simulink model "linear_flight_controller_payload"  (R2020a)
settings: Solver=FixedStepAuto  StartTime=0.0  StopTime=50  FixedStep=0.005  RelTol=1e-3
InitFcn:
  | flight_controller_payload_setup % Script to setup workspace
values from neighbouring files (symbols this model uses):
  C_Dx = 0.2    [PID_design_setup.m]    (also in flight_controller_payload_setup.m)
  C_Dz = 0.2    [PID_design_setup.m]    (also in flight_controller_payload_setup.m)
  C_px = 0.05    [flight_controller_payload_setup.m]
  C_pz = 0.05    [flight_controller_payload_setup.m]
  cbeta = 0.05    [flight_controller_payload_setup.m]
  dtheta_sp_max = 120*pi/180    (= 2.09439510239)    [flight_controller_payload_setup.m]
  dtheta_sp_min = -120*pi/180    (= -2.09439510239)    [flight_controller_payload_setup.m]
  dx_sp_max = 12    [flight_controller_payload_setup.m]
  dx_sp_min = -12    [flight_controller_payload_setup.m]
  dz_sp_max = 12    [flight_controller_payload_setup.m]
  dz_sp_min = -12    [flight_controller_payload_setup.m]
  g = -9.81    [PID_design_setup.m]    (also in flight_controller_payload_setup.m)
  I_yy = 0.235    [PID_design_setup.m]    (also in flight_controller_payload_setup.m)
  ki_dtheta = kp_dtheta*z_c    (= 0.1)    [PID_design_setup.m]
  kp_dtheta = 10^(K_dB/20)    [PID_design_setup.m]
  l = 1    [flight_controller_payload_setup.m]
  M = 4.5    [PID_design_setup.m]    (also in flight_controller_payload_setup.m)
  m = 2    [flight_controller_payload_setup.m]
  MM = [-1, 1 ... (first row only)    [flight_controller_payload_setup.m]    (also in flight_controller_setup.m = [-1/sqrt(2), -1)
  N_dtheta = Inf    (= inf)    [flight_controller_payload_setup.m]
  N_dx = 5*2*pi    (= 31.4159265359)    [flight_controller_payload_setup.m]
  N_dz = 5*2*pi    (= 31.4159265359)    [flight_controller_payload_setup.m]
  r = 0.49*1/sqrt(2)    [PID_design_setup.m]    (also in flight_controller_payload_setup.m)
  rho = 1.225    [PID_design_setup.m]    (also in flight_controller_payload_setup.m)
  sigma = 0    [flight_controller_payload_setup.m]
  tau = 0.07    [PID_design_setup.m]    (also in flight_controller_payload_setup.m)
  theta_sp_max = 30*pi/180    (= 0.523598775598)    [flight_controller_payload_setup.m]
  theta_sp_min = -30*pi/180    (= -0.523598775598)    [flight_controller_payload_setup.m]
  Ts_excite = 0    [flight_controller_payload_setup.m]
  Ts_mpc = 0.03    [flight_controller_payload_setup.m]
  u0 = -0.5*M*g*[1; 1]    [flight_controller_payload_setup.m]
  var_excite = 0    [flight_controller_payload_setup.m]
  x0 = zeros(nx,1)    [flight_controller_payload_setup.m]    (also in flight_controller_setup.m = zeros(6,1))
  x0_no_load = zeros(6,1)    [flight_controller_payload_setup.m]
undefined symbols (not defined in the file or in its folder): A_lin, B_lin, kd_dtheta, kd_dx, kd_dz, ki_dx, ki_dz, kp_dx, kp_dz, kp_theta, kp_x, kp_z
libraries: simulink x26, dspstat3 x8, mpclib x2
(part 3 of 3)

== system linear_flight_controller_payload/state space WITHOUT payload1/Angular rate controller1 ==
  note: PID to use auto tuning from simulink
  dtheta_sp : Inport
  X : Inport  Port=2
  Demux1 : Demux  Outputs=6
  Derivative : Derivative
  Gain : Gain  Gain=kd_dtheta
  I : Gain  Gain=ki_dtheta
  Integrator Limited : Integrator  LimitOutput=on  UpperSaturationLimit=10  LowerSaturationLimit=-10
  Low Pass Filter : TransferFcn  Denominator=[1/N_dtheta, 1]
  P : Gain  Gain=kp_dtheta
  PID Omega Controller : simulink/Continuous/PID Controller  Commented=on  Controller=PID  Form=Parallel  TimeDomain=Continuous-time  UseExternalTs=off  SampleTime=-1  IntegratorMethod=Forward Euler  FilterMethod=Forward Euler  ControllerParametersSource=internal  P=kp_dtheta  I=ki_dtheta  D=kd_dtheta  UseFilter=on  N=N_dtheta  TunerSelectOption=Transfer Function Based (PID Tuner App)  InitialConditionSource=internal  InitialConditionForIntegrator=0  InitialConditionForFilter=0  DifferentiatorICPrevScaledInput=0  ExternalReset=none  TrackingMode=off  Kt=1  LimitOutput=off  UpperSaturationLimit=inf  LowerSaturationLimit=-inf  LinearizeAsGain=on  AntiWindupMode=none  Kb=1  POutMin=[]  POutMax=[]  IOutMin=[]  IOutMax=[]  DOutMin=[]  DOutMax=[]  NOutMin=[]  NOutMax=[]  SumOutMin=[]  SumOutMax=[]  SaturationOutMin=[]  SaturationOutMax=[]  PParamMin=[]  PParamMax=[]  IParamMin=[]  IParamMax=[]  DParamMin=[]  DParamMax=[]  NParamMin=[]  NParamMax=[]  KbParamMin=[]  KbParamMax=[]  KtParamMin=[]  KtParamMax=[]  KbOutMin=[]  KbOutMax=[]  KtOutMin=[]  KtOutMax=[]  IntegratorOutMin=[]  IntegratorOutMax=[]  FilterOutMin=[]  FilterOutMax=[]  SumI1OutMin=[]  SumI1OutMax=[]  SumI2OutMin=[]  SumI2OutMax=[]  SumI3OutMin=[]  SumI3OutMax=[]  SumI4OutMin=[]  SumI4OutMax=[]  SumDOutMin=[]  SumDOutMax=[]  DifferentiatorOutMin=[]  DifferentiatorOutMax=[]  FilterDiffOutCoefMin=[]  FilterDiffOutCoefMax=[]  ReciprocalOutMin=[]  ReciprocalOutMax=[]  SumDenOutMin=[]  SumDenOutMax=[]  SumNumOutMin=[]  SumNumOutMax=[]  DivideOutMin=[]  DivideOutMax=[]  UdiffTsProdOutMin=[]  UdiffTsProdOutMax=[]  NTsProdOutMin=[]  NTsProdOutMax=[]  UintegralTsProdOutMin=[]  UintegralTsProdOutMax=[]  UngainTsProdOutMin=[]  UngainTsProdOutMax=[]  IntegratorContinuousStateAttributes=''  IntegratorStateMustResolveToSignalObject=off  IntegratorRTWStateStorageClass=Auto  FilterContinuousStateAttributes=''  FilterStateMustResolveToSignalObject=off  FilterRTWStateStorageClass=Auto  ParallelPVariant=InternalParameters  IdealPVariant=Disabled  IVariant=InternalParameters  DVariant=InternalParameters  IntegratorVariant=Continuous  SatVariant=Disabled  AWVariant=Passthrough  PCopyVariant=Disabled  TRVariant=Disabled  FdbkBlocksVariant=Forward  IdealPFdbkVariant=Disabled  SatFdbkVariant=Disabled  DerivativeFilterVariant=ContFilter  NVariant=InternalParameters  NCopyVariant=Disabled  FilterICVariant=InternalICsFilter  IntegratorICVariant=InternalICs  ExternalResetVariant=Disabled  TRSumVariant=Passthrough  SumFdbkVariant=Disabled  SumVariant=Sum_PID  TsampFilterVariant=InternalTs  TsampNgainVariant=Passthrough  TsampIntegralVariant=Passthrough
  Sum : Sum  Inputs=|+-
  Sum1 : Sum  Inputs=++-
  Sum2 : Sum  Inputs=++|
  delta_E : Outport
  wires:
  dtheta_sp/1 -> Sum/1
  Sum/1 -> P/1, Integrator Limited/1, PID Omega Controller/1
  Integrator Limited/1 -> I/1
  Derivative/1 -> Gain/1
  I/1 -> Sum1/2
  P/1 -> Sum1/1
  Gain/1 -> Sum1/3
  Sum1/1 -> Sum2/2
  Sum2/1 -> delta_E/1
  PID Omega Controller/1 -> Sum2/1
  Low Pass Filter/1 -> Derivative/1
  X/1 -> Demux1/1
  Demux1/6 -> Low Pass Filter/1, Sum/2  "dtheta"

== system linear_flight_controller_payload/state space WITHOUT payload1/Motor Mixing Algorithm1 ==
  delta_E : Inport
  delta_T : Inport  Port=2
  Mixing Matrix : Gain  Gain=MM  Multiplication=Matrix(K*u)
  Mux : Mux  Inputs=2
  Signal Specification : SignalSpecification  Dimensions=[2, 1]
  u : Outport  LockScale=on
  wires:
  delta_T/1 -> Mux/2
  delta_E/1 -> Mux/1
  Mixing Matrix/1 -> u/1
  Mux/1 -> Signal Specification/1
  Signal Specification/1 -> Mixing Matrix/1

== system linear_flight_controller_payload/state space WITHOUT payload1/Plant WITHOUT payload ==
  u : Inport  PortDimensions=[2, 1]
  Integrator : Integrator  Commented=on  InitialCondition=x0_no_load
  MATLAB Function1 : MATLAB Function  Commented=on  TreatAsAtomicUnit=on
  Motors : Subsystem
  Signal Specification : SignalSpecification  Dimensions=2
  State-Space : StateSpace  A=A_lin  B=B_lin  C=eye(6)  D=zeros(size(B_lin))  InitialCondition=zeros(6,1)
  parameters : Subsystem  Commented=on
  x : Outport
  wires:
  Motors/1(T) -> Signal Specification/1
  u/1 -> Motors/1(T_r)
  ? -> MATLAB Function1/2(u)
  Integrator/1 -> MATLAB Function1/1(x)
  parameters/1(parameters) -> MATLAB Function1/3(params)
  MATLAB Function1/1(dx) -> Integrator/1
  Signal Specification/1 -> State-Space/1
  State-Space/1 -> x/1

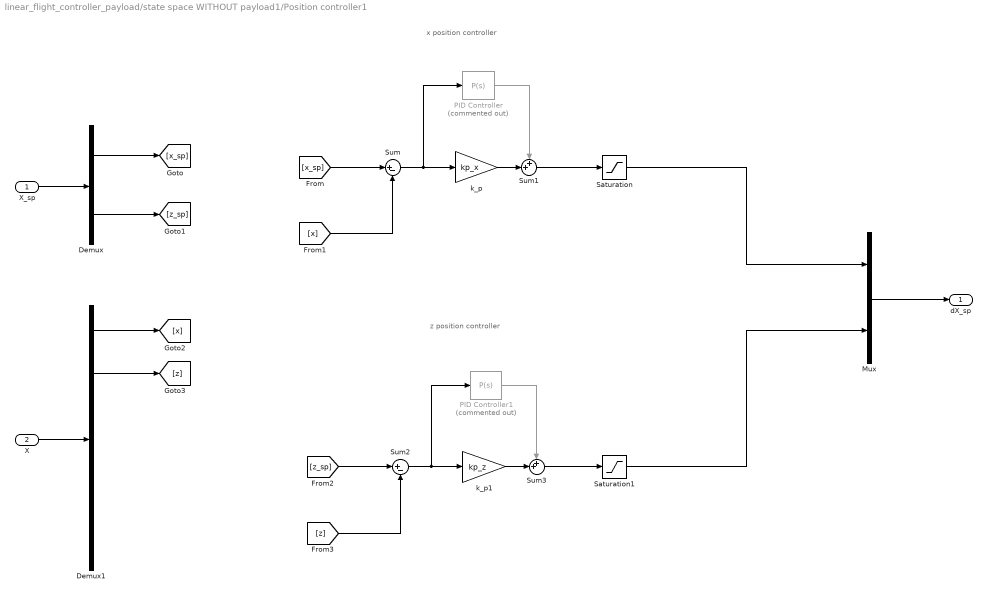
== system linear_flight_controller_payload/state space WITHOUT payload1/Position controller1 ==
  note: x position controller
  note: z position controller
  X_sp : Inport
  X : Inport  Port=2
  Demux : Demux  Outputs=2
  Demux1 : Demux  Outputs=6
  Mux : Mux  Inputs=2
  PID Controller : simulink/Continuous/PID Controller  Commented=on  Controller=P  Form=Parallel  TimeDomain=Continuous-time  UseExternalTs=off  SampleTime=-1  IntegratorMethod=Forward Euler  FilterMethod=Forward Euler  ControllerParametersSource=internal  P=20  I=1  D=0  UseFilter=on  N=100  TunerSelectOption=Transfer Function Based (PID Tuner App)  InitialConditionSource=internal  InitialConditionForIntegrator=0  InitialConditionForFilter=0  DifferentiatorICPrevScaledInput=0  ExternalReset=none  TrackingMode=off  Kt=1  LimitOutput=off  UpperSaturationLimit=inf  LowerSaturationLimit=-inf  LinearizeAsGain=on  AntiWindupMode=none  Kb=1  POutMin=[]  POutMax=[]  IOutMin=[]  IOutMax=[]  DOutMin=[]  DOutMax=[]  NOutMin=[]  NOutMax=[]  SumOutMin=[]  SumOutMax=[]  SaturationOutMin=[]  SaturationOutMax=[]  PParamMin=[]  PParamMax=[]  IParamMin=[]  IParamMax=[]  DParamMin=[]  DParamMax=[]  NParamMin=[]  NParamMax=[]  KbParamMin=[]  KbParamMax=[]  KtParamMin=[]  KtParamMax=[]  KbOutMin=[]  KbOutMax=[]  KtOutMin=[]  KtOutMax=[]  IntegratorOutMin=[]  IntegratorOutMax=[]  FilterOutMin=[]  FilterOutMax=[]  SumI1OutMin=[]  SumI1OutMax=[]  SumI2OutMin=[]  SumI2OutMax=[]  SumI3OutMin=[]  SumI3OutMax=[]  SumI4OutMin=[]  SumI4OutMax=[]  SumDOutMin=[]  SumDOutMax=[]  DifferentiatorOutMin=[]  DifferentiatorOutMax=[]  FilterDiffOutCoefMin=[]  FilterDiffOutCoefMax=[]  ReciprocalOutMin=[]  ReciprocalOutMax=[]  SumDenOutMin=[]  SumDenOutMax=[]  SumNumOutMin=[]  SumNumOutMax=[]  DivideOutMin=[]  DivideOutMax=[]  UdiffTsProdOutMin=[]  UdiffTsProdOutMax=[]  NTsProdOutMin=[]  NTsProdOutMax=[]  UintegralTsProdOutMin=[]  UintegralTsProdOutMax=[]  UngainTsProdOutMin=[]  UngainTsProdOutMax=[]  IntegratorContinuousStateAttributes=''  IntegratorStateMustResolveToSignalObject=off  IntegratorRTWStateStorageClass=Auto  FilterContinuousStateAttributes=''  FilterStateMustResolveToSignalObject=off  FilterRTWStateStorageClass=Auto  ParallelPVariant=InternalParameters  IdealPVariant=Disabled  IVariant=Disabled  DVariant=Disabled  IntegratorVariant=Disabled  SatVariant=Disabled  AWVariant=Disabled  PCopyVariant=Disabled  TRVariant=Disabled  FdbkBlocksVariant=Forward  IdealPFdbkVariant=Disabled  SatFdbkVariant=Disabled  DerivativeFilterVariant=Disabled  NVariant=Disabled  NCopyVariant=Disabled_SignalSpec  FilterICVariant=Disabled  IntegratorICVariant=Disabled  ExternalResetVariant=Disabled  TRSumVariant=Passthrough  SumFdbkVariant=Disabled  SumVariant=Passthrough_P  TsampFilterVariant=InternalTs  TsampNgainVariant=Passthrough  TsampIntegralVariant=Disabled_SignalSpec
  PID Controller1 : simulink/Continuous/PID Controller  Commented=on  Controller=P  Form=Parallel  TimeDomain=Continuous-time  UseExternalTs=off  SampleTime=-1  IntegratorMethod=Forward Euler  FilterMethod=Forward Euler  ControllerParametersSource=internal  P=1  I=1  D=0  UseFilter=on  N=100  TunerSelectOption=Transfer Function Based (PID Tuner App)  InitialConditionSource=internal  InitialConditionForIntegrator=0  InitialConditionForFilter=0  DifferentiatorICPrevScaledInput=0  ExternalReset=none  TrackingMode=off  Kt=1  LimitOutput=off  UpperSaturationLimit=inf  LowerSaturationLimit=-inf  LinearizeAsGain=on  AntiWindupMode=none  Kb=1  POutMin=[]  POutMax=[]  IOutMin=[]  IOutMax=[]  DOutMin=[]  DOutMax=[]  NOutMin=[]  NOutMax=[]  SumOutMin=[]  SumOutMax=[]  SaturationOutMin=[]  SaturationOutMax=[]  PParamMin=[]  PParamMax=[]  IParamMin=[]  IParamMax=[]  DParamMin=[]  DParamMax=[]  NParamMin=[]  NParamMax=[]  KbParamMin=[]  KbParamMax=[]  KtParamMin=[]  KtParamMax=[]  KbOutMin=[]  KbOutMax=[]  KtOutMin=[]  KtOutMax=[]  IntegratorOutMin=[]  IntegratorOutMax=[]  FilterOutMin=[]  FilterOutMax=[]  SumI1OutMin=[]  SumI1OutMax=[]  SumI2OutMin=[]  SumI2OutMax=[]  SumI3OutMin=[]  SumI3OutMax=[]  SumI4OutMin=[]  SumI4OutMax=[]  SumDOutMin=[]  SumDOutMax=[]  DifferentiatorOutMin=[]  DifferentiatorOutMax=[]  FilterDiffOutCoefMin=[]  FilterDiffOutCoefMax=[]  ReciprocalOutMin=[]  ReciprocalOutMax=[]  SumDenOutMin=[]  SumDenOutMax=[]  SumNumOutMin=[]  SumNumOutMax=[]  DivideOutMin=[]  DivideOutMax=[]  UdiffTsProdOutMin=[]  UdiffTsProdOutMax=[]  NTsProdOutMin=[]  NTsProdOutMax=[]  UintegralTsProdOutMin=[]  UintegralTsProdOutMax=[]  UngainTsProdOutMin=[]  UngainTsProdOutMax=[]  IntegratorContinuousStateAttributes=''  IntegratorStateMustResolveToSignalObject=off  IntegratorRTWStateStorageClass=Auto  FilterContinuousStateAttributes=''  FilterStateMustResolveToSignalObject=off  FilterRTWStateStorageClass=Auto  ParallelPVariant=InternalParameters  IdealPVariant=Disabled  IVariant=Disabled  DVariant=Disabled  IntegratorVariant=Disabled  SatVariant=Disabled  AWVariant=Disabled  PCopyVariant=Disabled  TRVariant=Disabled  FdbkBlocksVariant=Forward  IdealPFdbkVariant=Disabled  SatFdbkVariant=Disabled  DerivativeFilterVariant=Disabled  NVariant=Disabled  NCopyVariant=Disabled_SignalSpec  FilterICVariant=Disabled  IntegratorICVariant=Disabled  ExternalResetVariant=Disabled  TRSumVariant=Passthrough  SumFdbkVariant=Disabled  SumVariant=Passthrough_P  TsampFilterVariant=InternalTs  TsampNgainVariant=Passthrough  TsampIntegralVariant=Disabled_SignalSpec
  Saturation : Saturate  UpperLimit=dx_sp_max  LowerLimit=dx_sp_min
  Saturation1 : Saturate  UpperLimit=dz_sp_max  LowerLimit=dz_sp_min
  Sum : Sum  Inputs=|+-
  Sum1 : Sum  Inputs=++|
  Sum2 : Sum  Inputs=|+-
  Sum3 : Sum  Inputs=++|
  k_p : Gain  Gain=kp_x
  k_p1 : Gain  Gain=kp_z
  dX_sp : Outport
  wires:
  Sum/1 -> PID Controller/1, k_p/1
  k_p/1 -> Sum1/2
  PID Controller/1 -> Sum1/1
  X_sp/1 -> Demux/1
  Demux/2 -> [z_sp]
  Demux/1 -> [x_sp]
  X/1 -> Demux1/1
  Demux1/1 -> [x]
  Demux1/2 -> [z]
  [x_sp] -> Sum/1
  [x] -> Sum/2
  Sum2/1 -> PID Controller1/1, k_p1/1
  [z] -> Sum2/2
  [z_sp] -> Sum2/1
  PID Controller1/1 -> Sum3/1
  k_p1/1 -> Sum3/2
  Mux/1 -> dX_sp/1
  Sum1/1 -> Saturation/1
  Sum3/1 -> Saturation1/1
  Saturation1/1 -> Mux/2
  Saturation/1 -> Mux/1

== system linear_flight_controller_payload/state space WITHOUT payload1/Subsystem1 ==
  X : Inport
  Demux : Demux  Outputs=6
  theta : Outport
  wires:
  X/1 -> Demux/1
  Demux/3 -> theta/1

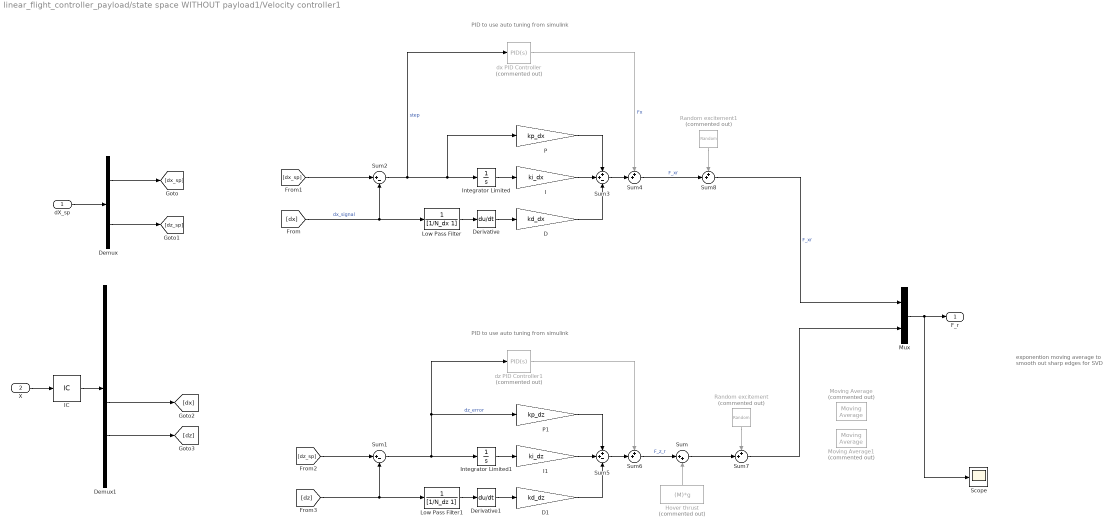
== system linear_flight_controller_payload/state space WITHOUT payload1/Velocity controller1 ==
  note: exponention moving average
      | to smooth out sharp edges for SVD
  note: PID to use auto tuning from simulink
  note: PID to use auto tuning from simulink
  dX_sp : Inport
  X : Inport  Port=2
  D : Gain  Gain=kd_dx
  D1 : Gain  Gain=kd_dz
  Demux : Demux  Outputs=2
  Demux1 : Demux  Outputs=6
  Derivative : Derivative
  Derivative1 : Derivative
  Hover thrust : Constant  Commented=on  Value=(M)*g
  I : Gain  Gain=ki_dx
  I1 : Gain  Gain=ki_dz
  IC : InitialCondition  Value=x0_no_load
  Integrator Limited : Integrator  LimitOutput=on  UpperSaturationLimit=10  LowerSaturationLimit=-10
  Integrator Limited1 : Integrator  LimitOutput=on  UpperSaturationLimit=10  LowerSaturationLimit=-10
  Low Pass Filter : TransferFcn  Denominator=[1/N_dx 1]
  Low Pass Filter1 : TransferFcn  Denominator=[1/N_dz 1]
  Moving Average : dspstat3/Moving Average  Commented=on  Method=Exponential weighting  ForgettingFactorPort=off  SpecifyWindowLength=on  WindowLength=4  ForgettingFactor=lambda  SimulateUsing=Code generation
  Moving Average1 : dspstat3/Moving Average  Commented=on  Method=Exponential weighting  ForgettingFactorPort=off  SpecifyWindowLength=on  WindowLength=4  ForgettingFactor=lambda  SimulateUsing=Code generation
  Mux : Mux  Inputs=2
  P : Gain  Gain=kp_dx
  P1 : Gain  Gain=kp_dz
  Random excitement : RandomNumber  Commented=on  Variance=var_excite  SampleTime=Ts_excite
  Random excitement1 : RandomNumber  Commented=on  Variance=var_excite  Seed=1  SampleTime=Ts_excite
  Scope : Scope
  Sum : Sum  Inputs=|++
  Sum1 : Sum  Inputs=|+-
  Sum2 : Sum  Inputs=|+-
  Sum3 : Sum  Inputs=++-
  Sum{4,6..8} (4 alike) : Sum  Inputs=++|
  Sum5 : Sum  Inputs=++-
  dx PID Controller : simulink/Continuous/PID Controller  Commented=on  Controller=PID  Form=Parallel  TimeDomain=Continuous-time  UseExternalTs=off  SampleTime=-1  IntegratorMethod=Forward Euler  FilterMethod=Forward Euler  ControllerParametersSource=internal  P=kp_dx  I=ki_dx  D=kd_dx  UseFilter=on  N=N_dx  TunerSelectOption=Transfer Function Based (PID Tuner App)  InitialConditionSource=internal  InitialConditionForIntegrator=0  InitialConditionForFilter=0  DifferentiatorICPrevScaledInput=0  ExternalReset=none  TrackingMode=off  Kt=1  LimitOutput=off  UpperSaturationLimit=inf  LowerSaturationLimit=-inf  LinearizeAsGain=on  AntiWindupMode=none  Kb=1  POutMin=[]  POutMax=[]  IOutMin=[]  IOutMax=[]  DOutMin=[]  DOutMax=[]  NOutMin=[]  NOutMax=[]  SumOutMin=[]  SumOutMax=[]  SaturationOutMin=[]  SaturationOutMax=[]  PParamMin=[]  PParamMax=[]  IParamMin=[]  IParamMax=[]  DParamMin=[]  DParamMax=[]  NParamMin=[]  NParamMax=[]  KbParamMin=[]  KbParamMax=[]  KtParamMin=[]  KtParamMax=[]  KbOutMin=[]  KbOutMax=[]  KtOutMin=[]  KtOutMax=[]  IntegratorOutMin=[]  IntegratorOutMax=[]  FilterOutMin=[]  FilterOutMax=[]  SumI1OutMin=[]  SumI1OutMax=[]  SumI2OutMin=[]  SumI2OutMax=[]  SumI3OutMin=[]  SumI3OutMax=[]  SumI4OutMin=[]  SumI4OutMax=[]  SumDOutMin=[]  SumDOutMax=[]  DifferentiatorOutMin=[]  DifferentiatorOutMax=[]  FilterDiffOutCoefMin=[]  FilterDiffOutCoefMax=[]  ReciprocalOutMin=[]  ReciprocalOutMax=[]  SumDenOutMin=[]  SumDenOutMax=[]  SumNumOutMin=[]  SumNumOutMax=[]  DivideOutMin=[]  DivideOutMax=[]  UdiffTsProdOutMin=[]  UdiffTsProdOutMax=[]  NTsProdOutMin=[]  NTsProdOutMax=[]  UintegralTsProdOutMin=[]  UintegralTsProdOutMax=[]  UngainTsProdOutMin=[]  UngainTsProdOutMax=[]  IntegratorContinuousStateAttributes=''  IntegratorStateMustResolveToSignalObject=off  IntegratorRTWStateStorageClass=Auto  FilterContinuousStateAttributes=''  FilterStateMustResolveToSignalObject=off  FilterRTWStateStorageClass=Auto  ParallelPVariant=InternalParameters  IdealPVariant=Disabled  IVariant=InternalParameters  DVariant=InternalParameters  IntegratorVariant=Continuous  SatVariant=Disabled  AWVariant=Passthrough  PCopyVariant=Disabled  TRVariant=Disabled  FdbkBlocksVariant=Forward  IdealPFdbkVariant=Disabled  SatFdbkVariant=Disabled  DerivativeFilterVariant=ContFilter  NVariant=InternalParameters  NCopyVariant=Disabled  FilterICVariant=InternalICsFilter  IntegratorICVariant=InternalICs  ExternalResetVariant=Disabled  TRSumVariant=Passthrough  SumFdbkVariant=Disabled  SumVariant=Sum_PID  TsampFilterVariant=InternalTs  TsampNgainVariant=Passthrough  TsampIntegralVariant=Passthrough
  dz PID Controller1 : simulink/Continuous/PID Controller  Commented=on  Controller=PID  Form=Parallel  TimeDomain=Continuous-time  UseExternalTs=off  SampleTime=-1  IntegratorMethod=Forward Euler  FilterMethod=Forward Euler  ControllerParametersSource=internal  P=kp_dz  I=ki_dz  D=kd_dz  UseFilter=on  N=N_dz  TunerSelectOption=Transfer Function Based (PID Tuner App)  InitialConditionSource=internal  InitialConditionForIntegrator=0  InitialConditionForFilter=0  DifferentiatorICPrevScaledInput=0  ExternalReset=none  TrackingMode=off  Kt=1  LimitOutput=off  UpperSaturationLimit=inf  LowerSaturationLimit=-inf  LinearizeAsGain=on  AntiWindupMode=none  Kb=1  POutMin=[]  POutMax=[]  IOutMin=[]  IOutMax=[]  DOutMin=[]  DOutMax=[]  NOutMin=[]  NOutMax=[]  SumOutMin=[]  SumOutMax=[]  SaturationOutMin=[]  SaturationOutMax=[]  PParamMin=[]  PParamMax=[]  IParamMin=[]  IParamMax=[]  DParamMin=[]  DParamMax=[]  NParamMin=[]  NParamMax=[]  KbParamMin=[]  KbParamMax=[]  KtParamMin=[]  KtParamMax=[]  KbOutMin=[]  KbOutMax=[]  KtOutMin=[]  KtOutMax=[]  IntegratorOutMin=[]  IntegratorOutMax=[]  FilterOutMin=[]  FilterOutMax=[]  SumI1OutMin=[]  SumI1OutMax=[]  SumI2OutMin=[]  SumI2OutMax=[]  SumI3OutMin=[]  SumI3OutMax=[]  SumI4OutMin=[]  SumI4OutMax=[]  SumDOutMin=[]  SumDOutMax=[]  DifferentiatorOutMin=[]  DifferentiatorOutMax=[]  FilterDiffOutCoefMin=[]  FilterDiffOutCoefMax=[]  ReciprocalOutMin=[]  ReciprocalOutMax=[]  SumDenOutMin=[]  SumDenOutMax=[]  SumNumOutMin=[]  SumNumOutMax=[]  DivideOutMin=[]  DivideOutMax=[]  UdiffTsProdOutMin=[]  UdiffTsProdOutMax=[]  NTsProdOutMin=[]  NTsProdOutMax=[]  UintegralTsProdOutMin=[]  UintegralTsProdOutMax=[]  UngainTsProdOutMin=[]  UngainTsProdOutMax=[]  IntegratorContinuousStateAttributes=''  IntegratorStateMustResolveToSignalObject=off  IntegratorRTWStateStorageClass=Auto  FilterContinuousStateAttributes=''  FilterStateMustResolveToSignalObject=off  FilterRTWStateStorageClass=Auto  ParallelPVariant=InternalParameters  IdealPVariant=Disabled  IVariant=InternalParameters  DVariant=InternalParameters  IntegratorVariant=Continuous  SatVariant=Disabled  AWVariant=Passthrough  PCopyVariant=Disabled  TRVariant=Disabled  FdbkBlocksVariant=Forward  IdealPFdbkVariant=Disabled  SatFdbkVariant=Disabled  DerivativeFilterVariant=ContFilter  NVariant=InternalParameters  NCopyVariant=Disabled  FilterICVariant=InternalICsFilter  IntegratorICVariant=InternalICs  ExternalResetVariant=Disabled  TRSumVariant=Passthrough  SumFdbkVariant=Disabled  SumVariant=Sum_PID  TsampFilterVariant=InternalTs  TsampNgainVariant=Passthrough  TsampIntegralVariant=Passthrough
  F_r : Outport
  wires:
  Derivative/1 -> D/1
  Sum3/1 -> Sum4/2
  Sum2/1 -> dx PID Controller/1, P/1, Integrator Limited/1  "step"
  I/1 -> Sum3/2
  Integrator Limited/1 -> I/1
  dx PID Controller/1 -> Sum4/1  "Fx"
  P/1 -> Sum3/1
  Low Pass Filter/1 -> Derivative/1
  D/1 -> Sum3/3
  P1/1 -> Sum5/1
  Integrator Limited1/1 -> I1/1
  dz PID Controller1/1 -> Sum6/1
  I1/1 -> Sum5/2
  Sum1/1 -> P1/1, dz PID Controller1/1, Integrator Limited1/1  "dz_error"
  Sum5/1 -> Sum6/2
  Low Pass Filter1/1 -> Derivative1/1
  Derivative1/1 -> D1/1
  D1/1 -> Sum5/3
  dX_sp/1 -> Demux/1
  [dx] -> Sum2/2, Low Pass Filter/1  "dx_signal"
  [dx_sp] -> Sum2/1
  Demux/1 -> [dx_sp]
  Demux/2 -> [dz_sp]
  [dz] -> Sum1/2, Low Pass Filter1/1
  [dz_sp] -> Sum1/1
  Demux1/4 -> [dx]
  Demux1/5 -> [dz]
  Sum6/1 -> Sum/1  "F_z_r"
  Hover thrust/1 -> Sum/2
  IC/1 -> Demux1/1
  X/1 -> IC/1
  Sum8/1 -> Mux/1  "F_xr"
  Sum7/1 -> Mux/2
  Mux/1 -> Scope/1, F_r/1
  Random excitement/1 -> Sum7/1
  Sum/1 -> Sum7/2
  Random excitement1/1 -> Sum8/1
  Sum4/1 -> Sum8/2  "F_xr"

== system linear_flight_controller_payload/Inner controllers and drone 2d1/Plant1/Motors ==
  T_r : Inport
  Gain : Gain  Gain=1/tau
  Integrator1 : Integrator  InitialCondition=u0
  Sum : Sum  Inputs=|+-
  T : Outport
  wires:
  Sum/1 -> Gain/1
  Gain/1 -> Integrator1/1  "dT"
  Integrator1/1 -> T/1, Sum/2  "T"
  T_r/1 -> Sum/1

== system linear_flight_controller_payload/Inner controllers and drone 2d1/Plant1/parameters ==
  " cbeta" : Constant  Value=cbeta
  " cbeta1" : Constant  Value=C_px
  " cbeta2" : Constant  Value=C_pz
  " rho" : Constant  Value=rho
  C_Dx : Constant  Value=C_Dx
  C_Dz : Constant  Value=C_Dz
  I_yy : Constant  Value=I_yy
  M : Constant  Value=M
  Mux : Mux  Inputs=12
  g : Constant  Value=g
  l : Constant  Value=l
  m : Constant  Value=m
  r : Constant  Value=r
  parameters : Outport
  wires:
  I_yy/1 -> Mux/2
  r/1 -> Mux/3
  Mux/1 -> parameters/1
  M/1 -> Mux/1
  C_Dx/1 -> Mux/5
  C_Dz/1 -> Mux/6
  g/1 -> Mux/4
  " rho"/1 -> Mux/7
  m/1 -> Mux/8
  l/1 -> Mux/9
  " cbeta"/1 -> Mux/10
  " cbeta1"/1 -> Mux/11
  " cbeta2"/1 -> Mux/12

== system linear_flight_controller_payload/MPC with linearised model WITHOUT payload1/Plant WITHOUT payload/Motors ==
  T_r : Inport
  Gain : Gain  Gain=1/tau
  Integrator1 : Integrator  InitialCondition=u0
  Sum : Sum  Inputs=|+-
  T : Outport
  wires:
  Sum/1 -> Gain/1
  Gain/1 -> Integrator1/1  "dT"
  Integrator1/1 -> T/1, Sum/2  "T"
  T_r/1 -> Sum/1

== system linear_flight_controller_payload/MPC with linearised model WITHOUT payload1/Plant WITHOUT payload/parameters ==
  " rho" : Constant  Value=rho
  C_Dx : Constant  Value=C_Dx
  C_Dz : Constant  Value=C_Dz
  I_yy : Constant  Value=I_yy
  M : Constant  Value=M
  Mux : Mux  Inputs=7
  g : Constant  Value=g
  r : Constant  Value=r
  parameters : Outport
  wires:
  I_yy/1 -> Mux/2
  r/1 -> Mux/3
  Mux/1 -> parameters/1
  M/1 -> Mux/1
  C_Dx/1 -> Mux/5
  C_Dz/1 -> Mux/6
  g/1 -> Mux/4
  " rho"/1 -> Mux/7

== system linear_flight_controller_payload/PID controllers WITHOUT payload/Plant WITHOUT payload/Motors ==
  T_r : Inport
  Gain : Gain  Gain=1/tau
  Integrator1 : Integrator  InitialCondition=u0
  Sum : Sum  Inputs=|+-
  T : Outport
  wires:
  Sum/1 -> Gain/1
  Gain/1 -> Integrator1/1  "dT"
  Integrator1/1 -> T/1, Sum/2  "T"
  T_r/1 -> Sum/1

== system linear_flight_controller_payload/PID controllers WITHOUT payload/Plant WITHOUT payload/parameters ==
  " rho" : Constant  Value=rho
  C_Dx : Constant  Value=C_Dx
  C_Dz : Constant  Value=C_Dz
  I_yy : Constant  Value=I_yy
  M : Constant  Value=M
  Mux : Mux  Inputs=7
  g : Constant  Value=g
  r : Constant  Value=r
  parameters : Outport
  wires:
  I_yy/1 -> Mux/2
  r/1 -> Mux/3
  Mux/1 -> parameters/1
  M/1 -> Mux/1
  C_Dx/1 -> Mux/5
  C_Dz/1 -> Mux/6
  g/1 -> Mux/4
  " rho"/1 -> Mux/7

== system linear_flight_controller_payload/PID controllers and Plant/Plant1/Motors ==
  T_r : Inport
  Gain : Gain  Gain=1/tau
  Integrator1 : Integrator  InitialCondition=u0
  Sum : Sum  Inputs=|+-
  T : Outport
  wires:
  Sum/1 -> Gain/1
  Gain/1 -> Integrator1/1  "dT"
  Integrator1/1 -> T/1, Sum/2  "T"
  T_r/1 -> Sum/1

== system linear_flight_controller_payload/PID controllers and Plant/Plant1/parameters ==
  " cbeta" : Constant  Value=cbeta
  " cbeta1" : Constant  Value=C_px
  " cbeta2" : Constant  Value=C_pz
  " rho" : Constant  Value=rho
  C_Dx : Constant  Value=C_Dx
  C_Dz : Constant  Value=C_Dz
  I_yy : Constant  Value=I_yy
  M : Constant  Value=M
  Mux : Mux  Inputs=12
  g : Constant  Value=g
  l : Constant  Value=l
  m : Constant  Value=m
  r : Constant  Value=r
  parameters : Outport
  wires:
  I_yy/1 -> Mux/2
  r/1 -> Mux/3
  Mux/1 -> parameters/1
  M/1 -> Mux/1
  C_Dx/1 -> Mux/5
  C_Dz/1 -> Mux/6
  g/1 -> Mux/4
  " rho"/1 -> Mux/7
  m/1 -> Mux/8
  l/1 -> Mux/9
  " cbeta"/1 -> Mux/10
  " cbeta1"/1 -> Mux/11
  " cbeta2"/1 -> Mux/12

== system linear_flight_controller_payload/state space WITHOUT payload1/Plant WITHOUT payload/Motors ==
  T_r : Inport
  Gain : Gain  Gain=1/tau
  Integrator1 : Integrator  InitialCondition=u0
  Sum : Sum  Inputs=|+-
  T : Outport
  wires:
  Sum/1 -> Gain/1
  Gain/1 -> Integrator1/1  "dT"
  Integrator1/1 -> T/1, Sum/2  "T"
  T_r/1 -> Sum/1

== system linear_flight_controller_payload/state space WITHOUT payload1/Plant WITHOUT payload/parameters ==
  " rho" : Constant  Value=rho
  C_Dx : Constant  Value=C_Dx
  C_Dz : Constant  Value=C_Dz
  I_yy : Constant  Value=I_yy
  M : Constant  Value=M
  Mux : Mux  Inputs=7
  g : Constant  Value=g
  r : Constant  Value=r
  parameters : Outport
  wires:
  I_yy/1 -> Mux/2
  r/1 -> Mux/3
  Mux/1 -> parameters/1
  M/1 -> Mux/1
  C_Dx/1 -> Mux/5
  C_Dz/1 -> Mux/6
  g/1 -> Mux/4
  " rho"/1 -> Mux/7

== matlab function linear_flight_controller_payload/MATLAB Function ==
  data: x input; x_noise output; sigma input
function x_noise = add_noise(x, sigma)
% Add normally distrubuted noise to signal
x_noise = x + sigma*randn(size(x));

end

== matlab function linear_flight_controller_payload/PID controllers and Plant/MATLAB Function1 ==
  data: F_r input; theta_sp output; delta_T output; theta input
function [theta_sp, delta_T]= inertial_to_body(F_r, theta)
%% Converts forces in inertial frame to body references (thrust and pitch reference)
% theta_sp = pitch set point
% delta_T = thrust reference
% F_r = [F_x_r, F_y_r], reference force vector in inertial frame

% NB: z is positive in down direction

delta_T = -0.5*F_r(2)/cos(theta);

theta_sp = -asin(min(max((F_r(1)/delta_T),-1),1)); % arcsine of bounded fraction. magnitude not larger than 1
% Linearised:
% theta_sp = -F_r(1)/delta_T; % magnitude not larger than 1
% theta_sp = max(min(theta_sp, pi/2), -pi/2);
end

== matlab function linear_flight_controller_payload/PID controllers and Plant/Plant1/MATLAB Function1 ==
  data: x input; u input; dx output; params input
function dx = drone_2D_payload(x,u,params)
    %% Differential equations for drone in 2D without a payload
    % dx: x_dot, time derivative of state vector
    % x: state vector [x, z, theta]
    % u: input vector
    % params: parameters for drone model
    
    % Parameters:
    M     = params(1); % Mass of drone body (at fulcrum)
    I_yy  = params(2); % Moment of inertia of drone body
    r     = params(3); % Distance from each rot`or force to COM of drone
    g     = params(4); % Acceleration due to gravity (always negative)
    C_Dx  = params(5); % Damping coef. of drone through air in x direction (f = cx*xdot)
    C_Dz  = params(6); % Damping coef. of drone in z direction (f = cy*zdot)
    rho   = params(7); % Air density
    
    m     = params(8); % Mass of suspended payload
    l     = params(9); % Length of suspended cable
    cbeta = params(10); % Damping coef of rotation about suspended link
    
    C_px  = params(11); % Damping coef. of payload through air in x direction (f = cx*xdot)
    C_pz  = params(12); % Damping coef. of payload in z direction (f = cy*zdot)   
    
    % States (extract notation so we can copy over from symbolic toolbox equations)
    X1 = x(1); % x
    X2 = x(2); % z
    X3 = x(3); % theta
    X4 = x(4); % beta
    X5 = x(5); % dx
    X6 = x(6); % dz
    X7 = x(7); % dtheta
    X8 = x(8); % dbeta
    
    % Inputs
    T1 = u(1);
    T2 = u(2);
    
    % System equations
    n = 8; % Number of states
    dx = zeros(n,1);
    
    dx(1,1) = x(5);
    dx(2,1) = x(6);
    dx(3,1) = x(7);
    dx(4,1) = x(8);
    
    dx(5,1) = (4*M*X8*cbeta*cos(X4) - 4*M*T1*l*sin(X3) - 4*M*T2*l*sin(X3) + 4*X8*cbeta*m*cos(X4) + 4*M*X8^2*l^2*m*sin(X4) - 4*T1*l*m*cos(X4)^2*sin(X3) - 4*T2*l*m*cos(X4)^2*sin(X3) + 4*T1*l*m*cos(X3)*cos(X4)*sin(X4) + 4*T2*l*m*cos(X3)*cos(X4)*sin(X4) - 2*C_Dx*M*X5*l*rho*abs(X5) - 2*C_Dx*X5*l*m*rho*abs(X5)*cos(X4)^2 + C_Dz*X6*l*m*rho*sin(2*X4)*abs(X6) + 2*C_px*M*X5*l*rho*cos(X4)^2*abs(X5 + X8*l*cos(X4)) + 2*C_pz*M*X8*l^2*rho*abs(X6 - X8*l*sin(X4))*cos(X4) - C_pz*M*X6*l*rho*abs(X6 - X8*l*sin(X4))*sin(2*X4) + 2*C_px*X5*l*m*rho*cos(X4)^2*abs(X5 + X8*l*cos(X4)) + 2*C_pz*X8*l^2*m*rho*abs(X6 - X8*l*sin(X4))*cos(X4) - C_pz*X6*l*m*rho*abs(X6 - X8*l*sin(X4))*sin(2*X4) + 2*C_px*M*X8*l^2*rho*cos(X4)^3*abs(X5 + X8*l*cos(X4)) - 2*C_pz*M*X8*l^2*rho*abs(X6 - X8*l*sin(X4))*cos(X4)^3 + 2*C_px*X8*l^2*m*rho*cos(X4)^3*abs(X5 + X8*l*cos(X4)) - 2*C_pz*X8*l^2*m*rho*abs(X6 - X8*l*sin(X4))*cos(X4)^3)/(4*M*l*(M + m));
    dx(6,1) = -(8*M^2*g*l + 8*M*T1*l*cos(X3) + 8*M*T2*l*cos(X3) + 8*M*X8*cbeta*sin(X4) + 4*T1*l*m*cos(X3) + 4*T2*l*m*cos(X3) + 8*X8*cbeta*m*sin(X4) - 4*T1*l*m*cos(X3 - 2*X4) - 4*T2*l*m*cos(X3 - 2*X4) + 8*M*g*l*m - 8*M*X8^2*l^2*m*cos(X4) - 2*C_pz*M*X6*l*rho*abs(X6 - X8*l*sin(X4)) - 2*C_pz*X6*l*m*rho*abs(X6 - X8*l*sin(X4)) + 4*C_Dz*M*X6*l*rho*abs(X6) + 2*C_Dz*X6*l*m*rho*abs(X6) - 2*C_Dz*X6*l*m*rho*cos(2*X4)*abs(X6) - 2*C_Dx*X5*l*m*rho*sin(2*X4)*abs(X5) + 2*C_px*M*X5*l*rho*sin(2*X4)*abs(X5 + X8*l*cos(X4)) + 2*C_pz*M*X6*l*rho*abs(X6 - X8*l*sin(X4))*cos(2*X4) + C_px*M*X8*l^2*rho*sin(X4)*abs(X5 + X8*l*cos(X4)) + 3*C_pz*M*X8*l^2*rho*abs(X6 - X8*l*sin(X4))*sin(X4) + 2*C_px*X5*l*m*rho*sin(2*X4)*abs(X5 + X8*l*cos(X4)) + 2*C_pz*X6*l*m*rho*abs(X6 - X8*l*sin(X4))*cos(2*X4) + C_px*X8*l^2*m*rho*sin(X4)*abs(X5 + X8*l*cos(X4)) + 3*C_pz*X8*l^2*m*rho*abs(X6 - X8*l*sin(X4))*sin(X4) + C_px*M*X8*l^2*rho*sin(3*X4)*abs(X5 + X8*l*cos(X4)) - C_pz*M*X8*l^2*rho*abs(X6 - X8*l*sin(X4))*sin(3*X4) + C_px*X8*l^2*m*rho*sin(3*X4)*abs(X5 + X8*l*cos(X4)) - C_pz*X8*l^2*m*rho*abs(X6 - X8*l*sin(X4))*sin(3*X4))/(8*M*l*(M + m));
    dx(7,1) = -(r*(T1 - T2))/I_yy;
    dx(8,1) = -(2*M*X8*cbeta + 2*X8*cbeta*m + 2*T1*l*m*cos(X3)*sin(X4) - 2*T1*l*m*cos(X4)*sin(X3) + 2*T2*l*m*cos(X3)*sin(X4) - 2*T2*l*m*cos(X4)*sin(X3) - C_pz*X6*l*m*rho*abs(X6 - X8*l*sin(X4))*sin(X4) + C_px*M*X8*l^2*rho*cos(X4)^2*abs(X5 + X8*l*cos(X4)) + C_pz*M*X8*l^2*rho*abs(X6 - X8*l*sin(X4))*sin(X4)^2 + C_px*X8*l^2*m*rho*cos(X4)^2*abs(X5 + X8*l*cos(X4)) - C_Dx*X5*l*m*rho*abs(X5)*cos(X4) + C_Dz*X6*l*m*rho*abs(X6)*sin(X4) + C_pz*X8*l^2*m*rho*abs(X6 - X8*l*sin(X4))*sin(X4)^2 + C_px*M*X5*l*rho*cos(X4)*abs(X5 + X8*l*cos(X4)) - C_pz*M*X6*l*rho*abs(X6 - X8*l*sin(X4))*sin(X4) + C_px*X5*l*m*rho*cos(X4)*abs(X5 + X8*l*cos(X4)))/(2*M*l^2*m);


end

== matlab function linear_flight_controller_payload/Inner controllers and drone 2d1/MATLAB Function ==
  data: F_r input; theta_sp output; delta_T output; theta input
function [theta_sp, delta_T]= inertial_to_body(F_r, theta)
%% Converts forces in inertial frame to body references (thrust and pitch reference)
% theta_sp = pitch set point
% delta_T = thrust reference
% F_r = [F_x_r, F_y_r], reference force vector in inertial frame

% NB: z is positive in down direction

delta_T = -0.5*F_r(2)/cos(theta);

theta_sp = -asin(min(max((F_r(1)/delta_T),-1),1)); % arcsine of bounded fraction. magnitude not larger than 1
% Linearised:
% theta_sp = -F_r(1)/delta_T; % magnitude not larger than 1
% theta_sp = max(min(theta_sp, pi/2), -pi/2);
end

== matlab function linear_flight_controller_payload/PID controllers WITHOUT payload/MATLAB Function1 ==
  data: F_r input; theta_sp output; delta_T output; theta input
function [theta_sp, delta_T]= inertial_to_body(F_r, theta)
%% Converts forces in inertial frame to body references (thrust and pitch reference)
% theta_sp = pitch set point
% delta_T = thrust reference
% F_r = [F_x_r, F_y_r], reference force vector in inertial frame

% NB: z is positive in down direction

delta_T = -0.5*F_r(2)/cos(theta);

theta_sp = -asin(min(max((F_r(1)/delta_T),-1),1)); % arcsine of bounded fraction. magnitude not larger than 1
% Linearised:
% theta_sp = -F_r(1)/delta_T; % magnitude not larger than 1
% theta_sp = max(min(theta_sp, pi/2), -pi/2);
end

== matlab function linear_flight_controller_payload/PID controllers WITHOUT payload/Plant WITHOUT payload/MATLAB Function1 ==
  data: x input; u input; dx output; params input
function dx = drone_2D(x,u,params)
    %% Differential equations for drone in 2D without a payload
    % dx: x_dot, time derivative of state vector
    % x: state vector [x, z, theta]
    % u: input vector
    % params: parameters for drone model
    
    % Parameters:
    M     = params(1); % Mass of drone body (at fulcrum)
    I_yy  = params(2); % Moment of inertia of drone body
    r     = params(3); % Distance from each rot`or force to COM of drone
    g     = params(4); % Acceleration due to gravity (always negative)
    C_Dx  = params(5); % Damping coef. of drone through air in x direction (f = cx*xdot)
    C_Dz  = params(6); % Damping coef. of drone in z direction (f = cy*zdot)
    rho   = params(7); % Air density
    
    % States (extract notation so we can copy over from symbolic toolbox equations)
    X1 = x(1); % x
    X2 = x(2); % z
    X3 = x(3); % theta
    X4 = x(4); % dx
    X5 = x(5); % dz
    X6 = x(6); % dtheta
    
    % Inputs
    T1 = u(1);
    T2 = u(2);
    
    % System equations
    dx = zeros(6,1);
    
    dx(1,1) = x(4);
    dx(2,1) = x(5);
    dx(3,1) = x(6);
    
    dx(4,1) = -(2*T1*sin(X3) + 2*T2*sin(X3) + C_Dx*X4*rho*abs(X4))/(2*M);
    dx(5,1) = -(2*M*g + 2*T1*cos(X3) + 2*T2*cos(X3) + C_Dz*X5*rho*abs(X5))/(2*M);
    dx(6,1) = -(T1*r - T2*r)/I_yy;
end

== matlab function linear_flight_controller_payload/MPC with linearised model WITHOUT payload1/MATLAB Function1 ==
  data: F_r input; theta_sp output; delta_T output; theta input
function [theta_sp, delta_T]= inertial_to_body(F_r, theta)
%% Converts forces in inertial frame to body references (thrust and pitch reference)
% theta_sp = pitch set point
% delta_T = thrust reference
% F_r = [F_x_r, F_y_r], reference force vector in inertial frame

% NB: z is positive in down direction

delta_T = -0.5*F_r(2)/cos(theta);

theta_sp = -asin(min(max((F_r(1)/delta_T),-1),1)); % arcsine of bounded fraction. magnitude not larger than 1
% Linearised:
% theta_sp = -F_r(1)/delta_T; % magnitude not larger than 1
% theta_sp = max(min(theta_sp, pi/2), -pi/2);
end

== matlab function linear_flight_controller_payload/MPC with linearised model WITHOUT payload1/Plant WITHOUT payload/MATLAB Function1 ==
  data: x input; u input; dx output; params input
function dx = drone_2D(x,u,params)
    %% Differential equations for drone in 2D without a payload
    % dx: x_dot, time derivative of state vector
    % x: state vector [x, z, theta]
    % u: input vector
    % params: parameters for drone model
    
    % Parameters:
    M     = params(1); % Mass of drone body (at fulcrum)
    I_yy  = params(2); % Moment of inertia of drone body
    r     = params(3); % Distance from each rot`or force to COM of drone
    g     = params(4); % Acceleration due to gravity (always negative)
    C_Dx  = params(5); % Damping coef. of drone through air in x direction (f = cx*xdot)
    C_Dz  = params(6); % Damping coef. of drone in z direction (f = cy*zdot)
    rho   = params(7); % Air density
    
    % States (extract notation so we can copy over from symbolic toolbox equations)
    X1 = x(1); % x
    X2 = x(2); % z
    X3 = x(3); % theta
    X4 = x(4); % dx
    X5 = x(5); % dz
    X6 = x(6); % dtheta
    
    % Inputs
    T1 = u(1);
    T2 = u(2);
    
    % System equations
    dx = zeros(6,1);
    
    dx(1,1) = x(4);
    dx(2,1) = x(5);
    dx(3,1) = x(6);
    
    dx(4,1) = -(2*T1*sin(X3) + 2*T2*sin(X3) + C_Dx*X4*rho*abs(X4))/(2*M);
    dx(5,1) = -(2*M*g + 2*T1*cos(X3) + 2*T2*cos(X3) + C_Dz*X5*rho*abs(X5))/(2*M);
    dx(6,1) = -(T1*r - T2*r)/I_yy;
end

== matlab function linear_flight_controller_payload/state space WITHOUT payload1/MATLAB Function1 ==
  data: F_r input; theta_sp output; delta_T output; theta input
function [theta_sp, delta_T]= inertial_to_body(F_r, theta)
%% Converts forces in inertial frame to body references (thrust and pitch reference)
% theta_sp = pitch set point
% delta_T = thrust reference
% F_r = [F_x_r, F_y_r], reference force vector in inertial frame

% NB: z is positive in down direction

delta_T = -0.5*F_r(2)/cos(theta);

theta_sp = -asin(min(max((F_r(1)/delta_T),-1),1)); % arcsine of bounded fraction. magnitude not larger than 1
% Linearised:
% theta_sp = -F_r(1)/delta_T; % magnitude not larger than 1
% theta_sp = max(min(theta_sp, pi/2), -pi/2);
end

== matlab function linear_flight_controller_payload/Inner controllers and drone 2d1/Plant1/MATLAB Function1 ==
  data: x input; u input; dx output; params input
function dx = drone_2D_payload(x,u,params)
    %% Differential equations for drone in 2D without a payload
    % dx: x_dot, time derivative of state vector
    % x: state vector [x, z, theta]
    % u: input vector
    % params: parameters for drone model
    
    % Parameters:
    M     = params(1); % Mass of drone body (at fulcrum)
    I_yy  = params(2); % Moment of inertia of drone body
    r     = params(3); % Distance from each rot`or force to COM of drone
    g     = params(4); % Acceleration due to gravity (always negative)
    C_Dx  = params(5); % Damping coef. of drone through air in x direction (f = cx*xdot)
    C_Dz  = params(6); % Damping coef. of drone in z direction (f = cy*zdot)
    rho   = params(7); % Air density
    
    m     = params(8); % Mass of suspended payload
    l     = params(9); % Length of suspended cable
    cbeta = params(10); % Damping coef of rotation about suspended link
    
    C_px  = params(11); % Damping coef. of payload through air in x direction (f = cx*xdot)
    C_pz  = params(12); % Damping coef. of payload in z direction (f = cy*zdot)   
    
    % States (extract notation so we can copy over from symbolic toolbox equations)
    X1 = x(1); % x
    X2 = x(2); % z
    X3 = x(3); % theta
    X4 = x(4); % beta
    X5 = x(5); % dx
    X6 = x(6); % dz
    X7 = x(7); % dtheta
    X8 = x(8); % dbeta
    
    % Inputs
    T1 = u(1);
    T2 = u(2);
    
    % System equations
    n = 8; % Number of states
    dx = zeros(n,1);
    
    dx(1,1) = x(5);
    dx(2,1) = x(6);
    dx(3,1) = x(7);
    dx(4,1) = x(8);
    
    dx(5,1) = (4*M*X8*cbeta*cos(X4) - 4*M*T1*l*sin(X3) - 4*M*T2*l*sin(X3) + 4*X8*cbeta*m*cos(X4) + 4*M*X8^2*l^2*m*sin(X4) - 4*T1*l*m*cos(X4)^2*sin(X3) - 4*T2*l*m*cos(X4)^2*sin(X3) + 4*T1*l*m*cos(X3)*cos(X4)*sin(X4) + 4*T2*l*m*cos(X3)*cos(X4)*sin(X4) - 2*C_Dx*M*X5*l*rho*abs(X5) - 2*C_Dx*X5*l*m*rho*abs(X5)*cos(X4)^2 + C_Dz*X6*l*m*rho*sin(2*X4)*abs(X6) + 2*C_px*M*X5*l*rho*cos(X4)^2*abs(X5 + X8*l*cos(X4)) + 2*C_pz*M*X8*l^2*rho*abs(X6 - X8*l*sin(X4))*cos(X4) - C_pz*M*X6*l*rho*abs(X6 - X8*l*sin(X4))*sin(2*X4) + 2*C_px*X5*l*m*rho*cos(X4)^2*abs(X5 + X8*l*cos(X4)) + 2*C_pz*X8*l^2*m*rho*abs(X6 - X8*l*sin(X4))*cos(X4) - C_pz*X6*l*m*rho*abs(X6 - X8*l*sin(X4))*sin(2*X4) + 2*C_px*M*X8*l^2*rho*cos(X4)^3*abs(X5 + X8*l*cos(X4)) - 2*C_pz*M*X8*l^2*rho*abs(X6 - X8*l*sin(X4))*cos(X4)^3 + 2*C_px*X8*l^2*m*rho*cos(X4)^3*abs(X5 + X8*l*cos(X4)) - 2*C_pz*X8*l^2*m*rho*abs(X6 - X8*l*sin(X4))*cos(X4)^3)/(4*M*l*(M + m));
    dx(6,1) = -(8*M^2*g*l + 8*M*T1*l*cos(X3) + 8*M*T2*l*cos(X3) + 8*M*X8*cbeta*sin(X4) + 4*T1*l*m*cos(X3) + 4*T2*l*m*cos(X3) + 8*X8*cbeta*m*sin(X4) - 4*T1*l*m*cos(X3 - 2*X4) - 4*T2*l*m*cos(X3 - 2*X4) + 8*M*g*l*m - 8*M*X8^2*l^2*m*cos(X4) - 2*C_pz*M*X6*l*rho*abs(X6 - X8*l*sin(X4)) - 2*C_pz*X6*l*m*rho*abs(X6 - X8*l*sin(X4)) + 4*C_Dz*M*X6*l*rho*abs(X6) + 2*C_Dz*X6*l*m*rho*abs(X6) - 2*C_Dz*X6*l*m*rho*cos(2*X4)*abs(X6) - 2*C_Dx*X5*l*m*rho*sin(2*X4)*abs(X5) + 2*C_px*M*X5*l*rho*sin(2*X4)*abs(X5 + X8*l*cos(X4)) + 2*C_pz*M*X6*l*rho*abs(X6 - X8*l*sin(X4))*cos(2*X4) + C_px*M*X8*l^2*rho*sin(X4)*abs(X5 + X8*l*cos(X4)) + 3*C_pz*M*X8*l^2*rho*abs(X6 - X8*l*sin(X4))*sin(X4) + 2*C_px*X5*l*m*rho*sin(2*X4)*abs(X5 + X8*l*cos(X4)) + 2*C_pz*X6*l*m*rho*abs(X6 - X8*l*sin(X4))*cos(2*X4) + C_px*X8*l^2*m*rho*sin(X4)*abs(X5 + X8*l*cos(X4)) + 3*C_pz*X8*l^2*m*rho*abs(X6 - X8*l*sin(X4))*sin(X4) + C_px*M*X8*l^2*rho*sin(3*X4)*abs(X5 + X8*l*cos(X4)) - C_pz*M*X8*l^2*rho*abs(X6 - X8*l*sin(X4))*sin(3*X4) + C_px*X8*l^2*m*rho*sin(3*X4)*abs(X5 + X8*l*cos(X4)) - C_pz*X8*l^2*m*rho*abs(X6 - X8*l*sin(X4))*sin(3*X4))/(8*M*l*(M + m));
    dx(7,1) = -(r*(T1 - T2))/I_yy;
    dx(8,1) = -(2*M*X8*cbeta + 2*X8*cbeta*m + 2*T1*l*m*cos(X3)*sin(X4) - 2*T1*l*m*cos(X4)*sin(X3) + 2*T2*l*m*cos(X3)*sin(X4) - 2*T2*l*m*cos(X4)*sin(X3) - C_pz*X6*l*m*rho*abs(X6 - X8*l*sin(X4))*sin(X4) + C_px*M*X8*l^2*rho*cos(X4)^2*abs(X5 + X8*l*cos(X4)) + C_pz*M*X8*l^2*rho*abs(X6 - X8*l*sin(X4))*sin(X4)^2 + C_px*X8*l^2*m*rho*cos(X4)^2*abs(X5 + X8*l*cos(X4)) - C_Dx*X5*l*m*rho*abs(X5)*cos(X4) + C_Dz*X6*l*m*rho*abs(X6)*sin(X4) + C_pz*X8*l^2*m*rho*abs(X6 - X8*l*sin(X4))*sin(X4)^2 + C_px*M*X5*l*rho*cos(X4)*abs(X5 + X8*l*cos(X4)) - C_pz*M*X6*l*rho*abs(X6 - X8*l*sin(X4))*sin(X4) + C_px*X5*l*m*rho*cos(X4)*abs(X5 + X8*l*cos(X4)))/(2*M*l^2*m);


end

== matlab function linear_flight_controller_payload/state space WITHOUT payload1/Plant WITHOUT payload/MATLAB Function1 ==
  data: x input; u input; dx output; params input
function dx = drone_2D(x,u,params)
    %% Differential equations for drone in 2D without a payload
    % dx: x_dot, time derivative of state vector
    % x: state vector [x, z, theta]
    % u: input vector
    % params: parameters for drone model
    
    % Parameters:
    M     = params(1); % Mass of drone body (at fulcrum)
    I_yy  = params(2); % Moment of inertia of drone body
    r     = params(3); % Distance from each rot`or force to COM of drone
    g     = params(4); % Acceleration due to gravity (always negative)
    C_Dx  = params(5); % Damping coef. of drone through air in x direction (f = cx*xdot)
    C_Dz  = params(6); % Damping coef. of drone in z direction (f = cy*zdot)
    rho   = params(7); % Air density
    
    % States (extract notation so we can copy over from symbolic toolbox equations)
    X1 = x(1); % x
    X2 = x(2); % z
    X3 = x(3); % theta
    X4 = x(4); % dx
    X5 = x(5); % dz
    X6 = x(6); % dtheta
    
    % Inputs
    T1 = u(1);
    T2 = u(2);
    
    % System equations
    dx = zeros(6,1);
    
    dx(1,1) = x(4);
    dx(2,1) = x(5);
    dx(3,1) = x(6);
    
    dx(4,1) = -(2*T1*sin(X3) + 2*T2*sin(X3) + C_Dx*X4*rho*abs(X4))/(2*M);
    dx(5,1) = -(2*M*g + 2*T1*cos(X3) + 2*T2*cos(X3) + C_Dz*X5*rho*abs(X5))/(2*M);
    dx(6,1) = -(T1*r - T2*r)/I_yy;
end
